simulink model "untitled"  (R2016b)
settings: Solver=VariableStepAuto  StartTime=0.0  StopTime=10.0  RelTol=1e-3
undefined symbols (not defined in the file or in its folder): Angular, Linear
libraries: robotlib x2, robotalgslib x1
settings Model: Creator=Utente  LastModifiedBy=Utente

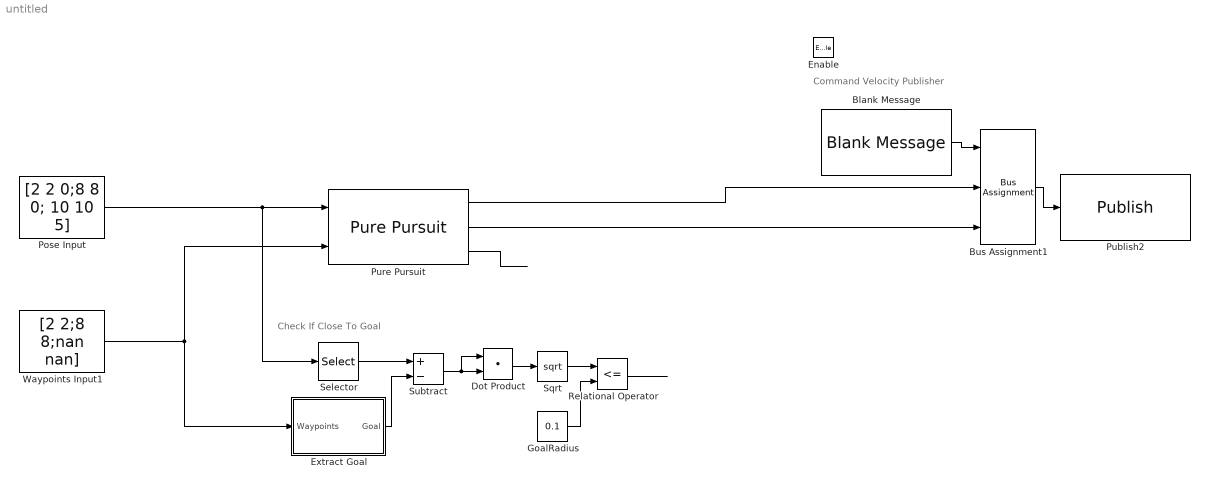
== system untitled ==
  note: Check If Close To Goal
  note: Command Velocity Publisher
  Enable : EnablePort
  " Extract Goal" : MATLAB Function  TreatAsAtomicUnit=on
  Blank Message : robotlib/Blank Message  SourceLibraryInfo=This block requires Robotics System Toolbox  messageType=geometry_msgs/Twist  SampleTime=inf
  Bus Assignment1 : BusAssignment  DialogController=Simulink.DDGSource_BusAssignment  AssignedSignals=Linear.X,Angular.Z
  Dot Product : DotProduct  InputSameDT=on  OutDataTypeStr=Inherit: Inherit via internal rule
  GoalRadius : Constant  Value=0.1
  Pose Input : Constant  Value=[2 2 0;8 8 0; 10 10 5]  OutDataTypeStr=double
  Publish2 : robotlib/Publish  SourceLibraryInfo=This block requires Robotics System Toolbox  topicSource=Select from ROS network  topic=/mobile_base/commands/velocity  messageType=geometry_msgs/Twist  messageQueueLength=105
  Pure Pursuit : robotalgslib/Pure Pursuit  DesiredLinearVelocity=0.3  MaxAngularVelocity=1.0  LookaheadDistance=2.0  TargetDirPort=on  SimulateUsing=Code generation
  Relational Operator : RelationalOperator  Operator=<=  OutDataTypeStr=boolean  RndMeth=Simplest
  Selector : Selector  InputPortWidth=3  IndexOptions=Index vector (dialog)  Indices=[1 2]  OutputSizes=1
  Sqrt : Sqrt  SaturateOnIntegerOverflow=on
  Subtract : Sum  Inputs=+-
  Waypoints Input1 : Constant  Value=[2 2;8 8;nan nan]  OutDataTypeStr=double
  wires:
  Pure Pursuit/3 -> ?
  Pure Pursuit/1 -> Bus Assignment1/2
  " Extract Goal"/1(Goal) -> Subtract/2
  Waypoints Input1/1 -> " Extract Goal"/1(Waypoints), Pure Pursuit/2
  Pose Input/1 -> Selector/1, Pure Pursuit/1
  Selector/1 -> Subtract/1
  Subtract/1 -> Dot Product/1, Dot Product/2
  Relational Operator/1 -> ?
  GoalRadius/1 -> Relational Operator/2
  Sqrt/1 -> Relational Operator/1
  Dot Product/1 -> Sqrt/1
  Pure Pursuit/2 -> Bus Assignment1/3
  Blank Message/1 -> Bus Assignment1/1
  Bus Assignment1/1 -> Publish2/1

== matlab function untitled/ Extract Goal ==
  data: Waypoints input; Goal output
function Goal = extractGoal(Waypoints)
%#codegen
b = isnan(Waypoints);
[rows,~] = find(b);
ridx = setdiff(1:size(Waypoints,1), sort(rows));
Goal = [Waypoints(ridx(end), 1) Waypoints(ridx(end), 2)];
